simulink library "INT_AFS_DD"  (R2016b)
settings: Solver=VariableStepAuto  StartTime=0.0  StopTime=10.0  RelTol=1e-3
settings Model: Creator=Colin  LastModifiedBy=Colin

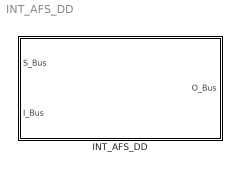
== system INT_AFS_DD ==
  INT_AFS_DD : Subsystem

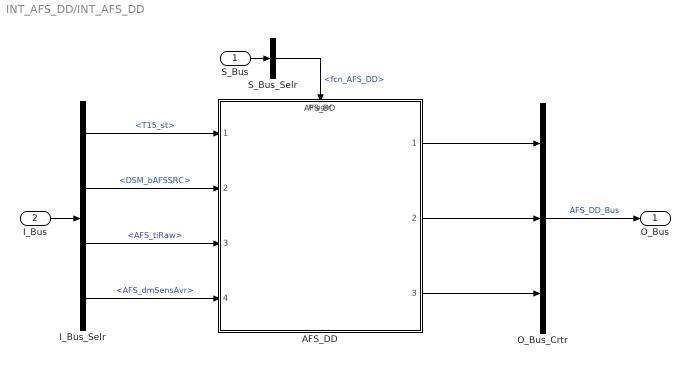
== system INT_AFS_DD/INT_AFS_DD ==
  S_Bus : Inport
  I_Bus : Inport  Port=2
  AFS_DD : ModelReference  ModelNameDialog=AFS_DD  SimulationMode=Normal  ModelReferenceVersion=1.59  TriggerPortName=function  TriggerPortTriggerType=function-call  TriggerPortStatesWhenEnabling=held
  I_Bus_Selr : BusSelector  OutputSignals=T15_st,DSM_bAFSSRC,AFS_tiRaw,AFS_dmSensAvr
  O_Bus_Crtr : BusCreator  Inputs=3
  S_Bus_Selr : BusSelector  OutputSignals=fcn_AFS_DD
  O_Bus : Outport
  wires:
  S_Bus_Selr/1 -> AFS_DD/Trigger  "<fcn_AFS_DD>"
  S_Bus/1 -> S_Bus_Selr/1
  I_Bus/1 -> I_Bus_Selr/1
  I_Bus_Selr/1 -> AFS_DD/1  "<T15_st>"
  I_Bus_Selr/2 -> AFS_DD/2  "<DSM_bAFSSRC>"
  I_Bus_Selr/3 -> AFS_DD/3  "<AFS_tiRaw>"
  I_Bus_Selr/4 -> AFS_DD/4  "<AFS_dmSensAvr>"
  O_Bus_Crtr/1 -> O_Bus/1  "AFS_DD_Bus"
  AFS_DD/1 -> O_Bus_Crtr/1
  AFS_DD/2 -> O_Bus_Crtr/2
  AFS_DD/3 -> O_Bus_Crtr/3
